simulink model "spring_pendulum"  (R2024b)
settings: Solver=ode4  StartTime=0.0  StopTime=100  FixedStep=2^-6  RelTol=1e-3
settings Model: Creator=zv53855  LastModifiedBy=zv53855

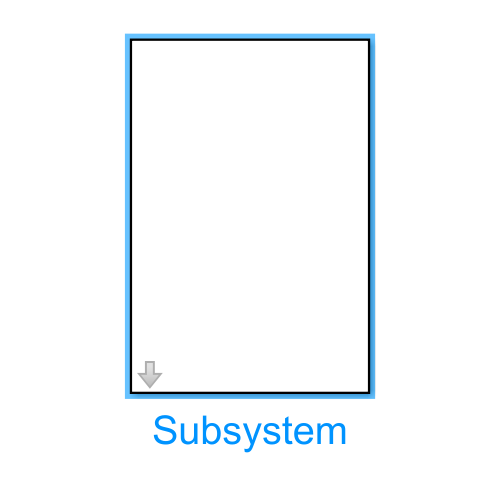
[thumbnail: Simulink's stored preview of the top-level diagram]
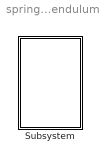
== system spring_pendulum ==
  Subsystem : Subsystem  mask{r1=1, r0=2, theta0=45*pi/180, theta1=12*pi/180, g=9.81, l=1.5, m=3, k=5}

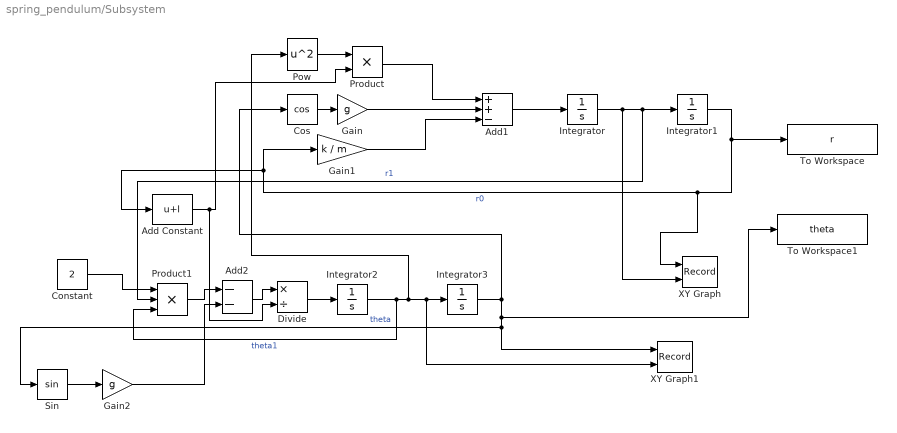
== system spring_pendulum/Subsystem ==
  Add Constant : Bias  Bias=l  SaturateOnIntegerOverflow=off
  Add1 : Sum  Inputs=++-
  Add2 : Sum  Inputs=--
  Constant : Constant  Value=2
  Cos : Trigonometry  Operator=cos
  Divide : Product  Inputs=*/
  Gain : Gain  Gain=g
  Gain1 : Gain  Gain=k / m
  Gain2 : Gain  Gain=g
  Integrator : Integrator  InitialCondition=r1
  Integrator1 : Integrator  InitialCondition=r0
  Integrator2 : Integrator  InitialCondition=theta1
  Integrator3 : Integrator  InitialCondition=theta0
  Pow : Math  Operator=square  SignedPower=on  RndMeth=Zero
  Product : Product
  Product1 : Product  Inputs=3
  Sin : Trigonometry
  To Workspace : ToWorkspace  VariableName=r  SampleTime=-1
  To Workspace1 : ToWorkspace  VariableName=theta  SampleTime=-1
  XY Graph : Record  FileSettingsInternal="{\"entries\":[{\"content\":{\"excelSettings\":{\"content\":{},\"type\":\"Streamout.ExcelSettings\"}},\"type\":\"Streamout.FileSettingStorage\",\"uuid\":\"\"}],\"packageUris\":[\"http:\\/\\/schema.mathworks.com\\/mf0\\/streamout_blocks\\/R2020a\"],\"version\":\"1.0\"}"  Layout=[1 1]  SignalsInternal="{\"entries\":[{\"content\":{\"signals\":[{\"content\":{\"blockPath\":[],\"dimensions\":[1],\"domain\":\"\",\"lineColor\":\"#a2142f\",\"plots\":[ 1 ],\"port\":1,\"sid\":[\"\"],\"signalID\":1,\"signalName\":\"r0\"},\"type\":\"RecordBlkView.Signal\",\"uuid\":\"\"},{\"content\":{\"blockPath\":[],\"dimensions\":[1],\"domain\":\"\",\"lineColor\":\"#139fff\",\"plots\":[ 1 ],\"port\":2,\"sid\":[\"\"],\"signalID\":2,\"signalName\":\"r1\"},\"type\":\"RecordBlkView.Signal\",\"uuid\":\"\"}]},\"type\":\"RecordBlkView.InputSignals\",\"uuid\":\"\"}],\"packageUris\":[\"http:\\/\\/schema.mathworks.com\\/mf0\\/streamout_blocks\\/R2020a\"],\"version\":\"1.0\"}"  VisualizationBindings="{\"xyplotplugin\":{\"info\":[{\"series\":[{\"bindingParametersList\":[{\"parameter\":\"X-Axis\",\"signalID\":1,\"signalName\":\"r0\"},{\"parameter\":\"Y-Axis\",\"signalID\":2,\"signalName\":\"r1\"}],\"seriesID\":0}],\"subplotID\":1}]}}"  CompatibilityTag=XY
  XY Graph1 : Record  FileSettingsInternal="{\"entries\":[{\"content\":{\"excelSettings\":{\"content\":{},\"type\":\"Streamout.ExcelSettings\"}},\"type\":\"Streamout.FileSettingStorage\",\"uuid\":\"\"}],\"packageUris\":[\"http:\\/\\/schema.mathworks.com\\/mf0\\/streamout_blocks\\/R2020a\"],\"version\":\"1.0\"}"  Layout=[1 1]  SignalsInternal="{\"entries\":[{\"content\":{\"signals\":[{\"content\":{\"blockPath\":[],\"dimensions\":[1],\"domain\":\"\",\"lineColor\":\"#a2142f\",\"plots\":[ 1 ],\"port\":1,\"sid\":[\"\"],\"signalID\":1,\"signalName\":\"theta\"},\"type\":\"RecordBlkView.Signal\",\"uuid\":\"\"},{\"content\":{\"blockPath\":[],\"dimensions\":[1],\"domain\":\"\",\"lineColor\":\"#139fff\",\"plots\":[ 1 ],\"port\":2,\"sid\":[\"\"],\"signalID\":2,\"signalName\":\"theta1\"},\"type\":\"RecordBlkView.Signal\",\"uuid\":\"\"}]},\"type\":\"RecordBlkView.InputSignals\",\"uuid\":\"\"}],\"packageUris\":[\"http:\\/\\/schema.mathworks.com\\/mf0\\/streamout_blocks\\/R2020a\"],\"version\":\"1.0\"}"  VisualizationBindings="{\"xyplotplugin\":{\"info\":[{\"series\":[{\"bindingParametersList\":[{\"parameter\":\"X-Axis\",\"signalID\":1,\"signalName\":\"theta\"},{\"parameter\":\"Y-Axis\",\"signalID\":2,\"signalName\":\"theta1\"}],\"seriesID\":0}],\"subplotID\":1}]}}"  CompatibilityTag=XY
  wires:
  Integrator1/1 -> To Workspace/1, XY Graph/1, Add Constant/1, Gain1/1  "r0"
  Add1/1 -> Integrator/1
  Product/1 -> Add1/1
  Integrator/1 -> XY Graph/2, Product1/2, Integrator1/1  "r1"
  Cos/1 -> Gain/1
  Integrator2/1 -> Product1/3, Pow/1, XY Graph1/2, Integrator3/1  "theta1"
  Integrator3/1 -> To Workspace1/1, XY Graph1/1, Sin/1, Cos/1  "theta"
  Gain1/1 -> Add1/3
  Gain/1 -> Add1/2
  Add Constant/1 -> Product/2, Divide/2
  Pow/1 -> Product/1
  Constant/1 -> Product1/1
  Sin/1 -> Gain2/1
  Product1/1 -> Add2/1
  Gain2/1 -> Add2/2
  Divide/1 -> Integrator2/1
  Add2/1 -> Divide/1
